simulink model "Test_Decoder_2_to_4"  (Simulink 8.1)
settings: Solver=ode45  StartTime=0.0  StopTime=len  RelTol=1e-3
libraries: commutil2 x2, Decoders_Lib x1
settings Model: Creator=N  LastModifiedBy=uzivatel
settings DataIOCC: LimitDataPoints=off  SignalLoggingSaveFormat=Dataset
settings OptimizationCC: ExpressionDepthLimit=128
settings DebuggingCC: UnderspecifiedInitializationDetection=Simplified  MergeDetectMultiDrivingBlocksExec=error  SolverPrmCheckMsg=none  FcnCallInpInsideContextMsg=EnableAllAsError  FrameProcessingCompatibilityMsg=error  StateNameClashWarn=none
settings HardwareCC: ProdBitPerPointer=64  ProdLargestAtomicFloat=Float  ProdIntDivRoundTo=Zero  ProdEndianess=LittleEndian  ProdHWDeviceType=Intel->x86-64 (Windows64)
settings ModelReferenceCC: PropagateSignalLabelsOutOfModel=on
settings GRTTargetCC: CodeReplacementLibrary=None  CombineOutputUpdateFcns=on  CPPClassGenCompliant=on  GRTInterface=off

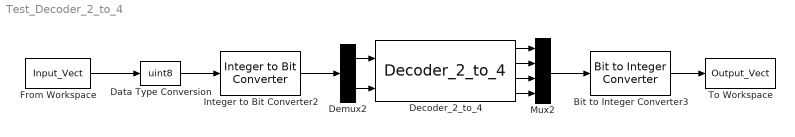
== system Test_Decoder_2_to_4 ==
  Bit to Integer Converter3 : commutil2/Bit to Integer Converter  nbits=4  bitOrder=MSB first  signedOutputValues=Unsigned  outDtype=uint8  outDtypeSigned=Inherit via internal rule
  Data Type Conversion : DataTypeConversion  OutDataTypeStr=uint8
  Decoder_2_to_4 : Decoders_Lib/Decoders_Lib/Decoder_2_to_4
  Demux2 : Demux  Outputs=2
  From Workspace : FromWorkspace  VariableName=Input_Vect  SampleTime=1  Interpolate=off  OutputAfterFinalValue=Holding final value
  Integer to Bit Converter2 : commutil2/Integer to Bit Converter  nbits=2  signedInputValues=Unsigned  bitOrder=MSB first  outDtype=boolean
  Mux2 : Mux
  To Workspace : ToWorkspace  VariableName=Output_Vect  SampleTime=1
  wires:
  Decoder_2_to_4/4 -> Mux2/4
  Decoder_2_to_4/3 -> Mux2/3
  Decoder_2_to_4/2 -> Mux2/2
  Decoder_2_to_4/1 -> Mux2/1
  Demux2/1 -> Decoder_2_to_4/1
  Demux2/2 -> Decoder_2_to_4/2
  Integer to Bit Converter2/1 -> Demux2/1
  Data Type Conversion/1 -> Integer to Bit Converter2/1
  Mux2/1 -> Bit to Integer Converter3/1
  From Workspace/1 -> Data Type Conversion/1
  Bit to Integer Converter3/1 -> To Workspace/1
